simulink model "saturn_thermal4"  (R2021a)
settings: Solver=ode23t  StartTime=0.0  StopTime=80000  MaxStep=1000  RelTol=1e-3
values from neighbouring files (symbols this model uses):
  Ab = L*l    [Data_ini_thermal_analysis4.m]    (also in Data_ini_thermal_analysis5.m)
  As = l*l    [Data_ini_thermal_analysis4.m]    (also in Data_ini_thermal_analysis5.m)
  D_st = 1224526    [Data_ini_thermal_analysis4.m]    (also in Data_ini_thermal_analysis5.m)
  ecc_sc = 0    [Data_ini_thermal_analysis4.m]    (also in Data_ini_thermal_analysis5.m)
  ecc_t = 0.0293    [Data_ini_thermal_analysis4.m]    (also in Data_ini_thermal_analysis5.m)
  incl_ax_s = deg2rad(26.73)    [Data_ini_thermal_analysis4.m]    (also in Data_ini_thermal_analysis5.m)
  incl_sc = deg2rad(90+45)    [Data_ini_thermal_analysis4.m]    (also in Data_ini_thermal_analysis5.m)
  incl_t = deg2rad(0.3485)    [Data_ini_thermal_analysis4.m]    (also in Data_ini_thermal_analysis5.m)
  mean_motion_sc = 2*pi/period_sc    [Data_ini_thermal_analysis4.m]    (also in Data_ini_thermal_analysis5.m)
  mean_motion_t = (2*pi)/period_t    (= 4.56068561416e-06)    [Data_ini_thermal_analysis4.m]    (also in Data_ini_thermal_analysis5.m)
  mean_r_s = 1.427*10^9    (= 1427000000)    [Data_ini_thermal_analysis4.m]    (also in Data_ini_thermal_analysis5.m)
  mu_s = 37931187    [Data_ini_thermal_analysis4.m]    (also in Data_ini_thermal_analysis5.m)
  mu_t = 8971.15    [Data_ini_thermal_analysis4.m]    (also in Data_ini_thermal_analysis5.m)
  period_s = 29.45*365*24*3600    (= 928735200)    [Data_ini_thermal_analysis4.m]    (also in Data_ini_thermal_analysis5.m)
  period_t = 15.945421*24*3600    (= 1377684.3744)    [Data_ini_thermal_analysis4.m]    (also in Data_ini_thermal_analysis5.m)
  R_s = diam_s/2    (= 60268)    [Data_ini_thermal_analysis4.m]    (also in Data_ini_thermal_analysis5.m)
  R_t = 2576    [Data_ini_thermal_analysis4.m]    (also in Data_ini_thermal_analysis5.m)
  semajax_sc = 1500+R_t    (= 4076)    [Data_ini_thermal_analysis4.m]    (also in Data_ini_thermal_analysis5.m)
  semajax_t = 1221830    [Data_ini_thermal_analysis4.m]    (also in Data_ini_thermal_analysis5.m)
libraries: fl_lib x283, nesl_utility x27
(part 1 of 3)
settings Model: Creator=dommy  LastModifiedBy=Riccardo
settings SolverCC: ZeroCrossAlgorithm=Adaptive
settings DebuggingCC: IgnoredZcDiagnostic=none

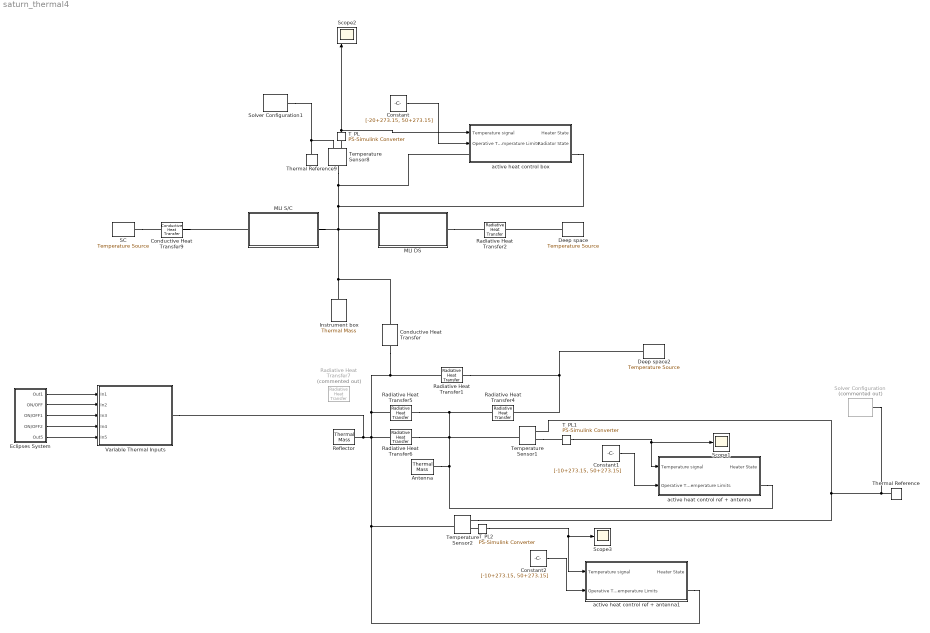
== system saturn_thermal4 ==
  Antenna : fl_lib/Thermal/Thermal Elements/Thermal Mass  mass=m_ant kg  sp_heat=cp_al J/kg/K  T_specify=on  T_priority=High  T=298 K  T_nominal_specify=off  T_nominal_unit=K  T_nominal_value=1  Q_specify=off  Q_priority=None  Q=0 W  Q_nominal_specify=off  Q_nominal_unit=W  Q_nominal_value=1
  Conductive Heat Transfer : fl_lib/Thermal/Thermal Elements/Conductive Heat Transfer  area=A_struc m^2  thickness=0.3 m  th_cond=k_al W/(m*K)  T_specify=off  T_priority=None  T=0 K  T_nominal_specify=off  T_nominal_unit=K  T_nominal_value=1  Q_specify=off  Q_priority=None  Q=0 W  Q_nominal_specify=off  Q_nominal_unit=W  Q_nominal_value=1
  Conductive Heat Transfer9 : fl_lib/Thermal/Thermal Elements/Conductive Heat Transfer  area=2*Ab m^2  thickness=s_kap m  th_cond=k_kap W/(m*K)  T_specify=off  T_priority=None  T=0 K  T_nominal_specify=off  T_nominal_unit=K  T_nominal_value=1  Q_specify=off  Q_priority=None  Q=0 W  Q_nominal_specify=off  Q_nominal_unit=W  Q_nominal_value=1
  Constant : Constant  Value=[-20+273.15, 50+273.15]
  Constant1 : Constant  Value=[-10+273.15, 50+273.15]
  Constant2 : Constant  Value=[-10+273.15, 50+273.15]
  Deep space : fl_lib/Thermal/Thermal Sources/Temperature Source  temperature=T_ds K
  Deep space2 : fl_lib/Thermal/Thermal Sources/Temperature Source  temperature=T_ds K
  Eclipses System : Subsystem
  Instrument box : fl_lib/Thermal/Thermal Elements/Thermal Mass  mass=25 kg  sp_heat=cp_al J/kg/K  T_specify=on  T_priority=High  T=298 K  T_nominal_specify=off  T_nominal_unit=K  T_nominal_value=1  Q_specify=off  Q_priority=None  Q=0 W  Q_nominal_specify=off  Q_nominal_unit=W  Q_nominal_value=1
  MLI DS : Subsystem
  MLI S/C : Subsystem
  Radiative Heat Transfer1 : fl_lib/Thermal/Thermal Elements/Radiative Heat Transfer  area=A_ref m^2  rad_tr_coeff=Gr_al W/(m^2*K^4)  T_specify=off  T_priority=None  T=0 K  T_nominal_specify=off  T_nominal_unit=K  T_nominal_value=1  Q_specify=off  Q_priority=None  Q=0 W  Q_nominal_specify=off  Q_nominal_unit=W  Q_nominal_value=1
      settings: SourceProductBaseCode=SS  InternalSimscapePortConfiguration="{\"Bottom\":[],\"Left\":[{\"id\":\"A\",\"label\":\"A\",\"type\":\"foundation.thermal.thermal\"}],\"Right\":[{\"id\":\"B\",\"label\":\"B\",\"type\":\"foundation.thermal.thermal\"}],\"Top\":[]}"
  Radiative Heat Transfer2 : fl_lib/Thermal/Thermal Elements/Radiative Heat Transfer  area=2*(Ab+As) m^2  rad_tr_coeff=Gr_kap W/(m^2*K^4)  T_specify=off  T_priority=None  T=0 K  T_nominal_specify=off  T_nominal_unit=K  T_nominal_value=1  Q_specify=off  Q_priority=None  Q=0 W  Q_nominal_specify=off  Q_nominal_unit=W  Q_nominal_value=1
      settings: SourceProductBaseCode=SS  InternalSimscapePortConfiguration="{\"Bottom\":[],\"Left\":[{\"id\":\"A\",\"label\":\"A\",\"type\":\"foundation.thermal.thermal\"}],\"Right\":[{\"id\":\"B\",\"label\":\"B\",\"type\":\"foundation.thermal.thermal\"}],\"Top\":[]}"
  Radiative Heat Transfer4 : fl_lib/Thermal/Thermal Elements/Radiative Heat Transfer  area=A_ant m^2  rad_tr_coeff=Gr_al W/(m^2*K^4)  T_specify=off  T_priority=None  T=0 K  T_nominal_specify=off  T_nominal_unit=K  T_nominal_value=1  Q_specify=off  Q_priority=None  Q=0 W  Q_nominal_specify=off  Q_nominal_unit=W  Q_nominal_value=1
      settings: SourceProductBaseCode=SS  InternalSimscapePortConfiguration="{\"Bottom\":[],\"Left\":[{\"id\":\"A\",\"label\":\"A\",\"type\":\"foundation.thermal.thermal\"}],\"Right\":[{\"id\":\"B\",\"label\":\"B\",\"type\":\"foundation.thermal.thermal\"}],\"Top\":[]}"
  Radiative Heat Transfer5 : fl_lib/Thermal/Thermal Elements/Radiative Heat Transfer  area=A_ref m^2  rad_tr_coeff=Gr_ra W/(m^2*K^4)  T_specify=off  T_priority=None  T=0 K  T_nominal_specify=off  T_nominal_unit=K  T_nominal_value=1  Q_specify=off  Q_priority=None  Q=0 W  Q_nominal_specify=off  Q_nominal_unit=W  Q_nominal_value=1
      settings: SourceProductBaseCode=SS  InternalSimscapePortConfiguration="{\"Bottom\":[],\"Left\":[{\"id\":\"A\",\"label\":\"A\",\"type\":\"foundation.thermal.thermal\"}],\"Right\":[{\"id\":\"B\",\"label\":\"B\",\"type\":\"foundation.thermal.thermal\"}],\"Top\":[]}"
  Radiative Heat Transfer6 : fl_lib/Thermal/Thermal Elements/Radiative Heat Transfer  area=A_ant m^2  rad_tr_coeff=Gr_ar W/(m^2*K^4)  T_specify=off  T_priority=None  T=0 K  T_nominal_specify=off  T_nominal_unit=K  T_nominal_value=1  Q_specify=off  Q_priority=None  Q=0 W  Q_nominal_specify=off  Q_nominal_unit=W  Q_nominal_value=1
      settings: SourceProductBaseCode=SS  InternalSimscapePortConfiguration="{\"Bottom\":[],\"Left\":[{\"id\":\"A\",\"label\":\"A\",\"type\":\"foundation.thermal.thermal\"}],\"Right\":[{\"id\":\"B\",\"label\":\"B\",\"type\":\"foundation.thermal.thermal\"}],\"Top\":[]}"
  Radiative Heat Transfer7 : fl_lib/Thermal/Thermal Elements/Radiative Heat Transfer  Commented=on  area=A_ref m^2  rad_tr_coeff=Gr_ra W/(m^2*K^4)  T_specify=off  T_priority=None  T=0 K  T_nominal_specify=off  T_nominal_unit=K  T_nominal_value=1  Q_specify=off  Q_priority=None  Q=0 W  Q_nominal_specify=off  Q_nominal_unit=W  Q_nominal_value=1
      settings: SourceProductBaseCode=SS  InternalSimscapePortConfiguration="{\"Bottom\":[],\"Left\":[{\"id\":\"A\",\"label\":\"A\",\"type\":\"foundation.thermal.thermal\"}],\"Right\":[{\"id\":\"B\",\"label\":\"B\",\"type\":\"foundation.thermal.thermal\"}],\"Top\":[]}"
  Reflector : fl_lib/Thermal/Thermal Elements/Thermal Mass  mass=m_ref kg  sp_heat=cp_al J/kg/K  T_specify=on  T_priority=High  T=298 K  T_nominal_specify=off  T_nominal_unit=K  T_nominal_value=1  Q_specify=off  Q_priority=None  Q=0 W  Q_nominal_specify=off  Q_nominal_unit=W  Q_nominal_value=1
  SC : fl_lib/Thermal/Thermal Sources/Temperature Source  temperature=300 K
  Scope1 : Scope
  Scope2 : Scope  NumInputPorts=3
  Scope3 : Scope
  Solver Configuration : nesl_utility/Solver Configuration  Commented=on  PhysicalDomain=network_engine_domain  SubClassName=solver  LeftPortType=input  RightPortType=generic  Tones=[]  Harmonics=[]  SimulateNoise=off  Profile=off  UseLocalSampling=off  EnableSwitchedLinearOptims=on  FrequencyDomain=off  UseCCode=off  RelTol=0.001  AbsTol=1e-06  MinStep=1e-09  ToWorkspace=off  RevertToSquareIcSolve=off  NumHomotopyIterations=100  PhasorMode=off  PhasorModeNumHarmonics=1  DoDC=off  ResidualTolerance=1e-09  UseLocalSolver=off  LocalSolverChoice=NE_BACKWARD_EULER_ADVANCER  LocalSolverSampleTime=0.001  DoFixedCost=off  MaxNonlinIter=3  MaxModeIter=2  ComputeImpulses=off  ImpulseIterations=2  LinearAlgebra=auto  EquationFormulation=NE_TIME_EF  DelaysMemoryBudget=1024  AutomaticFiltering=on  FilteringTimeConstant=0.001  PartitionStorageMethod=AS_NEEDED  PartitionMemoryBudget=1024  PartitionMethod=ROBUST
      settings: SourceProductBaseCode=PW,SS
  Solver Configuration1 : nesl_utility/Solver Configuration  PhysicalDomain=network_engine_domain  SubClassName=solver  LeftPortType=input  RightPortType=generic  Tones=[]  Harmonics=[]  SimulateNoise=off  Profile=off  UseLocalSampling=off  EnableSwitchedLinearOptims=on  FrequencyDomain=off  UseCCode=off  RelTol=0.001  AbsTol=1e-06  MinStep=1e-09  ToWorkspace=off  RevertToSquareIcSolve=off  NumHomotopyIterations=100  PhasorMode=off  PhasorModeNumHarmonics=1  DoDC=off  ResidualTolerance=1e-09  UseLocalSolver=off  LocalSolverChoice=NE_BACKWARD_EULER_ADVANCER  LocalSolverSampleTime=0.001  DoFixedCost=off  MaxNonlinIter=3  MaxModeIter=2  ComputeImpulses=off  ImpulseIterations=2  LinearAlgebra=auto  EquationFormulation=NE_TIME_EF  DelaysMemoryBudget=1024  AutomaticFiltering=on  FilteringTimeConstant=0.001  PartitionStorageMethod=AS_NEEDED  PartitionMemoryBudget=1024  PartitionMethod=ROBUST
      settings: SourceProductBaseCode=PW,SS
  T_PL : nesl_utility/PS-Simulink Converter  PhysicalDomain=network_engine_domain  SubClassName=ps_output  LeftPortType=input  RightPortType=output  PseudoPeriodic=off  Frequencies=[]  Unit=inherit  AffineConversion=off
      settings: SourceProductBaseCode=PW,SS
  T_PL1 : nesl_utility/PS-Simulink Converter  PhysicalDomain=network_engine_domain  SubClassName=ps_output  LeftPortType=input  RightPortType=output  PseudoPeriodic=off  Frequencies=[]  Unit=inherit  AffineConversion=off
      settings: SourceProductBaseCode=PW,SS
  T_PL2 : nesl_utility/PS-Simulink Converter  PhysicalDomain=network_engine_domain  SubClassName=ps_output  LeftPortType=input  RightPortType=output  PseudoPeriodic=off  Frequencies=[]  Unit=inherit  AffineConversion=off
      settings: SourceProductBaseCode=PW,SS
  Temperature Sensor1 : fl_lib/Thermal/Thermal Sensors/Temperature Sensor
  Temperature Sensor2 : fl_lib/Thermal/Thermal Sensors/Temperature Sensor
  Temperature Sensor8 : fl_lib/Thermal/Thermal Sensors/Temperature Sensor
  Thermal Reference : fl_lib/Thermal/Thermal Elements/Thermal Reference
  Thermal Reference9 : fl_lib/Thermal/Thermal Elements/Thermal Reference
  Variable Thermal Inputs : Subsystem
  active heat control box : Subsystem
  active heat control ref + antenna : Subsystem
  active heat control ref + antenna1 : Subsystem
  wires:
  Eclipses System/2(ON/OFF) -> Variable Thermal Inputs/2(In2)
  Eclipses System/3(ON/OFF1) -> Variable Thermal Inputs/3(In3)
  T_PL/1 -> Scope2/1, active heat control box/1(Temperature signal)
  Eclipses System/5(Out5) -> Variable Thermal Inputs/5(In5)
  Eclipses System/1(Out1) -> Variable Thermal Inputs/1(In1)
  Eclipses System/4(ON/OFF2) -> Variable Thermal Inputs/4(In4)
  T_PL1/1 -> Scope1/1, active heat control ref + antenna/1(Temperature signal)
  T_PL2/1 -> active heat control ref + antenna1/1(Temperature signal), Scope3/1
  Constant/1 -> active heat control box/2(Operative Temperature Limits)
  Constant1/1 -> active heat control ref + antenna/2(Operative Temperature Limits)
  Constant2/1 -> active heat control ref + antenna1/2(Operative Temperature Limits)
  connections:
  MLI DS/RConn1 -- Radiative Heat Transfer2/LConn1
  Temperature Sensor8/RConn1 -- Thermal Reference9/LConn1 -- Solver Configuration1/RConn1
  Temperature Sensor8/RConn2 -- T_PL/LConn1
  Deep space/LConn1 -- Radiative Heat Transfer2/RConn1
  Radiative Heat Transfer1/RConn1 -- Radiative Heat Transfer4/RConn1 -- Deep space2/LConn1
  SC/LConn1 -- Conductive Heat Transfer9/LConn1
  Conductive Heat Transfer9/RConn1 -- MLI S/C/RConn1
  Antenna/LConn1 -- Radiative Heat Transfer5/RConn1 -- Radiative Heat Transfer4/LConn1 -- Radiative Heat Transfer6/LConn1 -- Temperature Sensor1/LConn1 -- active heat control ref + antenna/RConn1
  Temperature Sensor1/RConn2 -- T_PL1/LConn1
  Thermal Reference/LConn1 -- Temperature Sensor2/RConn1 -- Temperature Sensor1/RConn1 -- Solver Configuration/RConn1
  Temperature Sensor2/RConn2 -- T_PL2/LConn1
  Instrument box/LConn1 -- Conductive Heat Transfer/RConn1 -- active heat control box/RConn1 -- active heat control box/LConn1 -- Temperature Sensor8/LConn1 -- MLI S/C/LConn1 -- MLI DS/LConn1
  Reflector/LConn1 -- Variable Thermal Inputs/RConn1 -- Radiative Heat Transfer6/RConn1 -- Conductive Heat Transfer/LConn1 -- Radiative Heat Transfer1/LConn1 -- Radiative Heat Transfer5/LConn1 -- Temperature Sensor2/LConn1 -- active heat control ref + antenna1/RConn1

== system saturn_thermal4/Eclipses System ==
  Add : Sum
  Constant : Constant  Value=0
  Saturn-Titan-SC : Subsystem
  Sun-Saturn-Titan : Subsystem
  Sun-Titan-SC : Subsystem
  Out1 : Outport
  ON/OFF : Outport  Port=2
  ON/OFF1 : Outport  Port=3
  ON/OFF2 : Outport  Port=4
  Out5 : Outport  Port=5
  wires:
  Sun-Titan-SC/1(ON/OFF) -> ON/OFF1/1, Add/2
  Constant/1 -> Out5/1
  Saturn-Titan-SC/1(ON/OFF) -> ON/OFF2/1
  Sun-Saturn-Titan/1(ON/OFF) -> ON/OFF/1, Add/1
  Add/1 -> Out1/1

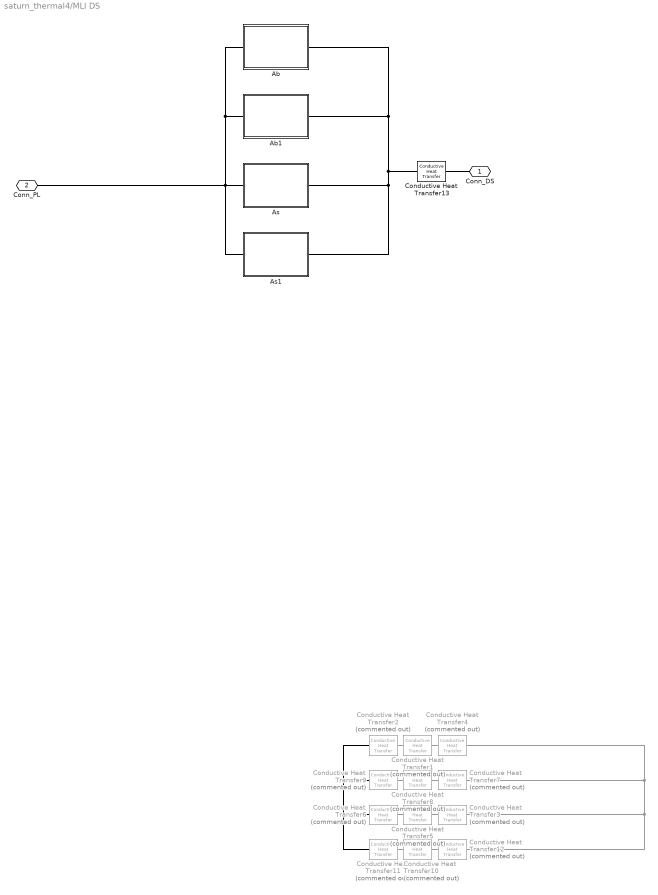
== system saturn_thermal4/MLI DS ==
  Ab : Subsystem
  Ab1 : Subsystem
  As : Subsystem
  As1 : Subsystem
  Conductive Heat Transfer1 : fl_lib/Thermal/Thermal Elements/Conductive Heat Transfer  Commented=on  area=As m^2  thickness=s_tfe_out m  th_cond=k_tfe W/(m*K)  T_specify=off  T_priority=None  T=0 K  T_nominal_specify=off  T_nominal_unit=K  T_nominal_value=1  Q_specify=off  Q_priority=None  Q=0 W  Q_nominal_specify=off  Q_nominal_unit=W  Q_nominal_value=1
  Conductive Heat Transfer10 : fl_lib/Thermal/Thermal Elements/Conductive Heat Transfer  Commented=on  area=As m^2  thickness=s_tfe_out m  th_cond=k_tfe W/(m*K)  T_specify=off  T_priority=None  T=0 K  T_nominal_specify=off  T_nominal_unit=K  T_nominal_value=1  Q_specify=off  Q_priority=None  Q=0 W  Q_nominal_specify=off  Q_nominal_unit=W  Q_nominal_value=1
  Conductive Heat Transfer{2,4,11..12} (4 alike) : fl_lib/Thermal/Thermal Elements/Conductive Heat Transfer  Commented=on  area=As m^2  thickness=s_al m  th_cond=k_al W/(m*K)  T_specify=off  T_priority=None  T=0 K  T_nominal_specify=off  T_nominal_unit=K  T_nominal_value=1  Q_specify=off  Q_priority=None  Q=0 W  Q_nominal_specify=off  Q_nominal_unit=W  Q_nominal_value=1
  Conductive Heat Transfer13 : fl_lib/Thermal/Thermal Elements/Conductive Heat Transfer  area=2*(Ab+As) m^2  thickness=s_kap m  th_cond=k_kap W/(m*K)  T_specify=off  T_priority=None  T=0 K  T_nominal_specify=off  T_nominal_unit=K  T_nominal_value=1  Q_specify=off  Q_priority=None  Q=0 W  Q_nominal_specify=off  Q_nominal_unit=W  Q_nominal_value=1
  Conductive Heat Transfer{3,6..7,9} (4 alike) : fl_lib/Thermal/Thermal Elements/Conductive Heat Transfer  Commented=on  area=Ab m^2  thickness=s_al m  th_cond=k_al W/(m*K)  T_specify=off  T_priority=None  T=0 K  T_nominal_specify=off  T_nominal_unit=K  T_nominal_value=1  Q_specify=off  Q_priority=None  Q=0 W  Q_nominal_specify=off  Q_nominal_unit=W  Q_nominal_value=1
  Conductive Heat Transfer5 : fl_lib/Thermal/Thermal Elements/Conductive Heat Transfer  Commented=on  area=Ab m^2  thickness=s_tfe_out m  th_cond=k_tfe W/(m*K)  T_specify=off  T_priority=None  T=0 K  T_nominal_specify=off  T_nominal_unit=K  T_nominal_value=1  Q_specify=off  Q_priority=None  Q=0 W  Q_nominal_specify=off  Q_nominal_unit=W  Q_nominal_value=1
  Conductive Heat Transfer8 : fl_lib/Thermal/Thermal Elements/Conductive Heat Transfer  Commented=on  area=Ab m^2  thickness=s_tfe_out m  th_cond=k_tfe W/(m*K)  T_specify=off  T_priority=None  T=0 K  T_nominal_specify=off  T_nominal_unit=K  T_nominal_value=1  Q_specify=off  Q_priority=None  Q=0 W  Q_nominal_specify=off  Q_nominal_unit=W  Q_nominal_value=1
  Conn_DS : PMIOPort  Side=Right
  "Conn_PL\t" : PMIOPort  Port=2  Side=Left
  connections:
  Conductive Heat Transfer7/RConn1 -- Conductive Heat Transfer3/RConn1 -- Conductive Heat Transfer12/RConn1 -- Conductive Heat Transfer4/RConn1
  Conductive Heat Transfer11/RConn1 -- Conductive Heat Transfer10/LConn1
  Conductive Heat Transfer12/LConn1 -- Conductive Heat Transfer10/RConn1
  Conductive Heat Transfer6/RConn1 -- Conductive Heat Transfer5/LConn1
  Conductive Heat Transfer3/LConn1 -- Conductive Heat Transfer5/RConn1
  Conductive Heat Transfer7/LConn1 -- Conductive Heat Transfer8/RConn1
  Conductive Heat Transfer9/RConn1 -- Conductive Heat Transfer8/LConn1
  Conductive Heat Transfer4/LConn1 -- Conductive Heat Transfer1/RConn1
  Conductive Heat Transfer2/RConn1 -- Conductive Heat Transfer1/LConn1
  Conductive Heat Transfer9/LConn1 -- Conductive Heat Transfer11/LConn1 -- Conductive Heat Transfer6/LConn1 -- Conductive Heat Transfer2/LConn1
  "Conn_PL\t"/RConn1 -- Ab/LConn1 -- Ab1/LConn1 -- As/LConn1 -- As1/LConn1
  Conn_DS/RConn1 -- Conductive Heat Transfer13/RConn1
  Conductive Heat Transfer13/LConn1 -- Ab/RConn1 -- Ab1/RConn1 -- As/RConn1 -- As1/RConn1

== system saturn_thermal4/MLI S//C ==
  Ab : Subsystem
  Ab1 : Subsystem
  Conductive Heat Transfer1 : fl_lib/Thermal/Thermal Elements/Conductive Heat Transfer  Commented=on  area=As m^2  thickness=s_tfe_out m  th_cond=k_tfe W/(m*K)  T_specify=off  T_priority=None  T=0 K  T_nominal_specify=off  T_nominal_unit=K  T_nominal_value=1  Q_specify=off  Q_priority=None  Q=0 W  Q_nominal_specify=off  Q_nominal_unit=W  Q_nominal_value=1
  Conductive Heat Transfer10 : fl_lib/Thermal/Thermal Elements/Conductive Heat Transfer  Commented=on  area=As m^2  thickness=s_tfe_out m  th_cond=k_tfe W/(m*K)  T_specify=off  T_priority=None  T=0 K  T_nominal_specify=off  T_nominal_unit=K  T_nominal_value=1  Q_specify=off  Q_priority=None  Q=0 W  Q_nominal_specify=off  Q_nominal_unit=W  Q_nominal_value=1
  Conductive Heat Transfer{2,4,11..12} (4 alike) : fl_lib/Thermal/Thermal Elements/Conductive Heat Transfer  Commented=on  area=As m^2  thickness=s_al m  th_cond=k_al W/(m*K)  T_specify=off  T_priority=None  T=0 K  T_nominal_specify=off  T_nominal_unit=K  T_nominal_value=1  Q_specify=off  Q_priority=None  Q=0 W  Q_nominal_specify=off  Q_nominal_unit=W  Q_nominal_value=1
  Conductive Heat Transfer{3,6..7,9} (4 alike) : fl_lib/Thermal/Thermal Elements/Conductive Heat Transfer  Commented=on  area=Ab m^2  thickness=s_al m  th_cond=k_al W/(m*K)  T_specify=off  T_priority=None  T=0 K  T_nominal_specify=off  T_nominal_unit=K  T_nominal_value=1  Q_specify=off  Q_priority=None  Q=0 W  Q_nominal_specify=off  Q_nominal_unit=W  Q_nominal_value=1
  Conductive Heat Transfer5 : fl_lib/Thermal/Thermal Elements/Conductive Heat Transfer  Commented=on  area=Ab m^2  thickness=s_tfe_out m  th_cond=k_tfe W/(m*K)  T_specify=off  T_priority=None  T=0 K  T_nominal_specify=off  T_nominal_unit=K  T_nominal_value=1  Q_specify=off  Q_priority=None  Q=0 W  Q_nominal_specify=off  Q_nominal_unit=W  Q_nominal_value=1
  Conductive Heat Transfer8 : fl_lib/Thermal/Thermal Elements/Conductive Heat Transfer  Commented=on  area=Ab m^2  thickness=s_tfe_out m  th_cond=k_tfe W/(m*K)  T_specify=off  T_priority=None  T=0 K  T_nominal_specify=off  T_nominal_unit=K  T_nominal_value=1  Q_specify=off  Q_priority=None  Q=0 W  Q_nominal_specify=off  Q_nominal_unit=W  Q_nominal_value=1
  Conn_S/C : PMIOPort  Side=Right
  "Conn_PL\t" : PMIOPort  Port=2  Side=Left
  connections:
  Ab1/RConn1 -- Ab/RConn1 -- Conn_S/C/RConn1
  Ab1/LConn1 -- Ab/LConn1 -- "Conn_PL\t"/RConn1
  Conductive Heat Transfer2/LConn1 -- Conductive Heat Transfer6/LConn1 -- Conductive Heat Transfer11/LConn1 -- Conductive Heat Transfer9/LConn1
  Conductive Heat Transfer2/RConn1 -- Conductive Heat Transfer1/LConn1
  Conductive Heat Transfer4/LConn1 -- Conductive Heat Transfer1/RConn1
  Conductive Heat Transfer9/RConn1 -- Conductive Heat Transfer8/LConn1
  Conductive Heat Transfer7/LConn1 -- Conductive Heat Transfer8/RConn1
  Conductive Heat Transfer3/LConn1 -- Conductive Heat Transfer5/RConn1
  Conductive Heat Transfer6/RConn1 -- Conductive Heat Transfer5/LConn1
  Conductive Heat Transfer12/LConn1 -- Conductive Heat Transfer10/RConn1
  Conductive Heat Transfer11/RConn1 -- Conductive Heat Transfer10/LConn1
  Conductive Heat Transfer4/RConn1 -- Conductive Heat Transfer12/RConn1 -- Conductive Heat Transfer3/RConn1 -- Conductive Heat Transfer7/RConn1

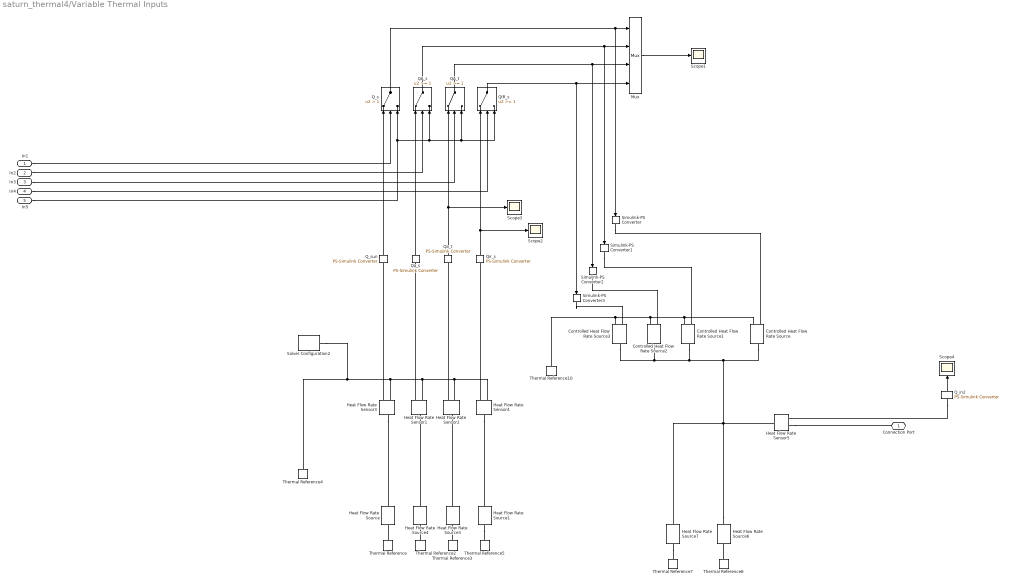
== system saturn_thermal4/Variable Thermal Inputs ==
  In1 : Inport
  In2 : Inport  Port=2
  In3 : Inport  Port=3
  In4 : Inport  Port=4
  In5 : Inport  Port=5
  Controlled Heat Flow Rate Source{,1..3} (4 alike) : fl_lib/Thermal/Thermal Sources/Controlled Heat Flow Rate Source
  Heat Flow Rate Sensor{1..5} (5 alike) : fl_lib/Thermal/Thermal Sensors/Heat Flow Rate Sensor
      settings: SourceProductBaseCode=SS
  Heat Flow Rate Source : fl_lib/Thermal/Thermal Sources/Heat Flow Rate Source  heat_flow=Qs_s W
      settings: SourceProductBaseCode=SS  InternalSimscapePortConfiguration="{\"Bottom\":[],\"Left\":[{\"id\":\"B\",\"label\":\"B\",\"type\":\"foundation.thermal.thermal\"}],\"Right\":[{\"id\":\"A\",\"label\":\"A\",\"type\":\"foundation.thermal.thermal\"}],\"Top\":[]}"
  Heat Flow Rate Source1 : fl_lib/Thermal/Thermal Sources/Heat Flow Rate Source  heat_flow=Qir_s W
      settings: SourceProductBaseCode=SS  InternalSimscapePortConfiguration="{\"Bottom\":[],\"Left\":[{\"id\":\"B\",\"label\":\"B\",\"type\":\"foundation.thermal.thermal\"}],\"Right\":[{\"id\":\"A\",\"label\":\"A\",\"type\":\"foundation.thermal.thermal\"}],\"Top\":[]}"
  Heat Flow Rate Source3 : fl_lib/Thermal/Thermal Sources/Heat Flow Rate Source  heat_flow=Qa_t W
      settings: SourceProductBaseCode=SS  InternalSimscapePortConfiguration="{\"Bottom\":[],\"Left\":[{\"id\":\"B\",\"label\":\"B\",\"type\":\"foundation.thermal.thermal\"}],\"Right\":[{\"id\":\"A\",\"label\":\"A\",\"type\":\"foundation.thermal.thermal\"}],\"Top\":[]}"
  Heat Flow Rate Source4 : fl_lib/Thermal/Thermal Sources/Heat Flow Rate Source  heat_flow=Qa_s W
      settings: SourceProductBaseCode=SS  InternalSimscapePortConfiguration="{\"Bottom\":[],\"Left\":[{\"id\":\"B\",\"label\":\"B\",\"type\":\"foundation.thermal.thermal\"}],\"Right\":[{\"id\":\"A\",\"label\":\"A\",\"type\":\"foundation.thermal.thermal\"}],\"Top\":[]}"
  Heat Flow Rate Source6 : fl_lib/Thermal/Thermal Sources/Heat Flow Rate Source  heat_flow=45 W
      settings: SourceProductBaseCode=SS  InternalSimscapePortConfiguration="{\"Bottom\":[],\"Left\":[{\"id\":\"B\",\"label\":\"B\",\"type\":\"foundation.thermal.thermal\"}],\"Right\":[{\"id\":\"A\",\"label\":\"A\",\"type\":\"foundation.thermal.thermal\"}],\"Top\":[]}"
  Heat Flow Rate Source7 : fl_lib/Thermal/Thermal Sources/Heat Flow Rate Source  heat_flow=Qir_t W
      settings: SourceProductBaseCode=SS  InternalSimscapePortConfiguration="{\"Bottom\":[],\"Left\":[{\"id\":\"B\",\"label\":\"B\",\"type\":\"foundation.thermal.thermal\"}],\"Right\":[{\"id\":\"A\",\"label\":\"A\",\"type\":\"foundation.thermal.thermal\"}],\"Top\":[]}"
  Mux : Mux
  QA_s : Switch  Threshold=1
  QA_t : Switch  Threshold=1
  QIR_s : Switch  Threshold=1
  Q_in2 : nesl_utility/PS-Simulink Converter  PhysicalDomain=network_engine_domain  SubClassName=ps_output  LeftPortType=input  RightPortType=output  PseudoPeriodic=off  Frequencies=[]  Unit=inherit  AffineConversion=off
      settings: SourceProductBaseCode=PW,SS
  Q_s : Switch  Criteria=u2 > Threshold  Threshold=1
  Q_sun : nesl_utility/PS-Simulink Converter  PhysicalDomain=network_engine_domain  SubClassName=ps_output  LeftPortType=input  RightPortType=output  PseudoPeriodic=off  Frequencies=[]  Unit=inherit  AffineConversion=off
      settings: SourceProductBaseCode=PW,SS
  Qa_s : nesl_utility/PS-Simulink Converter  PhysicalDomain=network_engine_domain  SubClassName=ps_output  LeftPortType=input  RightPortType=output  PseudoPeriodic=off  Frequencies=[]  Unit=inherit  AffineConversion=off
      settings: SourceProductBaseCode=PW,SS
  Qa_t : nesl_utility/PS-Simulink Converter  PhysicalDomain=network_engine_domain  SubClassName=ps_output  LeftPortType=input  RightPortType=output  PseudoPeriodic=off  Frequencies=[]  Unit=inherit  AffineConversion=off
      settings: SourceProductBaseCode=PW,SS
  Qir_s : nesl_utility/PS-Simulink Converter  PhysicalDomain=network_engine_domain  SubClassName=ps_output  LeftPortType=input  RightPortType=output  PseudoPeriodic=off  Frequencies=[]  Unit=inherit  AffineConversion=off
      settings: SourceProductBaseCode=PW,SS
  Scope{1..4} (4 alike) : Scope
  Simulink-PS Converter{,1..3} (4 alike) : nesl_utility/Simulink-PS Converter  PhysicalDomain=network_engine_domain  SubClassName=ps_input  LeftPortType=input  RightPortType=output  PseudoPeriodic=off  Frequencies=[]  NoiseDistribution=none  NoiseParameters=[]  Unit=1  AffineConversion=off  FilteringAndDerivatives=provide  SimscapeFilterOrder=1  InputFilterTimeConstant=0.001  UdotUserProvided=0
      settings: SourceProductBaseCode=PW,SS
  Solver Configuration2 : nesl_utility/Solver Configuration  PhysicalDomain=network_engine_domain  SubClassName=solver  LeftPortType=input  RightPortType=generic  Tones=[]  Harmonics=[]  SimulateNoise=off  Profile=off  UseLocalSampling=off  EnableSwitchedLinearOptims=on  FrequencyDomain=off  UseCCode=off  RelTol=0.001  AbsTol=1e-06  MinStep=1e-09  ToWorkspace=off  RevertToSquareIcSolve=off  NumHomotopyIterations=100  PhasorMode=off  PhasorModeNumHarmonics=1  DoDC=off  ResidualTolerance=1e-09  UseLocalSolver=off  LocalSolverChoice=NE_BACKWARD_EULER_ADVANCER  LocalSolverSampleTime=0.001  DoFixedCost=off  MaxNonlinIter=3  MaxModeIter=2  ComputeImpulses=off  ImpulseIterations=2  LinearAlgebra=auto  EquationFormulation=NE_TIME_EF  DelaysMemoryBudget=1024  AutomaticFiltering=on  FilteringTimeConstant=0.001  PartitionStorageMethod=AS_NEEDED  PartitionMemoryBudget=1024  PartitionMethod=ROBUST
      settings: SourceProductBaseCode=PW,SS
  Thermal Reference{,2..5,7..8,10} (8 alike) : fl_lib/Thermal/Thermal Elements/Thermal Reference
  Connection Port : PMIOPort  Side=Right
  wires:
  QA_t/1 -> Simulink-PS Converter2/1, Mux/3
  In5/1 -> QA_s/3, QIR_s/3, QA_t/3, Q_s/3
  Qa_s/1 -> QA_s/1
  QIR_s/1 -> Simulink-PS Converter3/1, Mux/4
  QA_s/1 -> Simulink-PS Converter1/1, Mux/2
  Qa_t/1 -> Scope3/1, QA_t/1
  Q_sun/1 -> Q_s/1
  Q_s/1 -> Simulink-PS Converter/1, Mux/1
  Qir_s/1 -> QIR_s/1, Scope2/1
  Mux/1 -> Scope1/1
  In4/1 -> QIR_s/2
  In2/1 -> QA_s/2
  In1/1 -> Q_s/2
  In3/1 -> QA_t/2
  Q_in2/1 -> Scope4/1
  connections:
  Thermal Reference4/LConn1 -- Solver Configuration2/RConn1 -- Heat Flow Rate Sensor3/RConn2 -- Heat Flow Rate Sensor1/RConn2 -- Heat Flow Rate Sensor2/RConn2 -- Heat Flow Rate Sensor4/RConn2
  Thermal Reference8/LConn1 -- Heat Flow Rate Source6/RConn1
  Heat Flow Rate Sensor1/LConn1 -- Heat Flow Rate Source4/LConn1
  Heat Flow Rate Source4/RConn1 -- Thermal Reference2/LConn1
  Thermal Reference10/LConn1 -- Controlled Heat Flow Rate Source3/RConn2 -- Controlled Heat Flow Rate Source/RConn2 -- Controlled Heat Flow Rate Source1/RConn2 -- Controlled Heat Flow Rate Source2/RConn2
  Thermal Reference3/LConn1 -- Heat Flow Rate Source3/RConn1
  Heat Flow Rate Source1/RConn1 -- Thermal Reference5/LConn1
  Heat Flow Rate Sensor2/RConn1 -- Qa_t/LConn1
  Thermal Reference/LConn1 -- Heat Flow Rate Source/RConn1
  Simulink-PS Converter1/RConn1 -- Controlled Heat Flow Rate Source1/RConn1
  Simulink-PS Converter2/RConn1 -- Controlled Heat Flow Rate Source2/RConn1
  Simulink-PS Converter3/RConn1 -- Controlled Heat Flow Rate Source3/RConn1
  Heat Flow Rate Sensor1/RConn1 -- Qa_s/LConn1
  Heat Flow Rate Sensor4/RConn1 -- Qir_s/LConn1
  Heat Flow Rate Source7/RConn1 -- Thermal Reference7/LConn1
  Simulink-PS Converter/RConn1 -- Controlled Heat Flow Rate Source/RConn1
  Heat Flow Rate Sensor3/RConn1 -- Q_sun/LConn1
  Heat Flow Rate Sensor4/LConn1 -- Heat Flow Rate Source1/LConn1
  Heat Flow Rate Sensor2/LConn1 -- Heat Flow Rate Source3/LConn1
  Heat Flow Rate Sensor3/LConn1 -- Heat Flow Rate Source/LConn1
  Q_in2/LConn1 -- Heat Flow Rate Sensor5/RConn1
  Heat Flow Rate Source6/LConn1 -- Heat Flow Rate Sensor5/LConn1 -- Heat Flow Rate Source7/LConn1 -- Controlled Heat Flow Rate Source/LConn1 -- Controlled Heat Flow Rate Source3/LConn1 -- Controlled Heat Flow Rate Source2/LConn1 -- Controlled Heat Flow Rate Source1/LConn1
  Heat Flow Rate Sensor5/RConn2 -- Connection Port/RConn1

== system saturn_thermal4/active heat control box ==
  Temperature signal : Inport
  Operative Temperature Limits : Inport  Port=2
  Constant : Constant  Value=0
  Demux : Demux  Outputs=2
  Heater Watts : Constant  Value=50
  Subsystem : Subsystem
  Subsystem1 : Subsystem
      settings: PortSchema="{\"entries\":[{\"content\":{\"sides\":[{\"content\":{\"connectorIds\":[\"In1\",\"LConn1\",\"In2\",\"In3\"]},\"type\":\"ConnectorPlacement.EquallySpacedRectSide\",\"uuid\":\"bd26e488-957e-4768-8c8f-f592c40ec45a\"},{\"content\":{\"connectorIds\":[\"Out1\"],\"side\":\"RIGHT\"},\"type\":\"ConnectorPlacement.EquallySpacedRectSide\",\"uuid\":\"e3290ae6-0dd6-4908-9dc2-c69eb2f26011\"},{\"content\":{\"connectorIds\":[],\"side\":\"TOP\"},\"type\":\"ConnectorPlacement.EquallySpacedRectSide\",\"uuid\":\"6f74d5de-8d2d-4ebd-b7f8-350d8117613a\"}]},\"type\":\"ConnectorPlacement.EquallySpacedConnector\",\"uuid\":\"06df4fc0-1d31-4bf7-986e-18508187f506\"}],\"packageUris\":[\"http://schema.mathworks.com/mf0/Connector/R2020b\"],\"version\":\"1.0\"}"
  heat block : PMIOPort  Side=Left
  Heater Sink : PMIOPort  Port=2  Side=Right
  Heater State : Outport
  Radiator State : Outport  Port=2
  wires:
  Temperature signal/1 -> Subsystem1/1(signal), Subsystem/1(signal)
  Operative Temperature Limits/1 -> Demux/1
  Demux/1 -> Subsystem/2(reference)
  Demux/2 -> Subsystem1/2(reference)
  Constant/1 -> Subsystem/4(off case), Subsystem1/3(off case)
  Heater Watts/1 -> Subsystem/3(on case)
  Subsystem/1(Output) -> Heater State/1
  Subsystem1/1(Output) -> Radiator State/1
  connections:
  heat block/RConn1 -- Subsystem1/LConn1
  Heater Sink/RConn1 -- Subsystem/RConn1

== system saturn_thermal4/active heat control ref + antenna ==
  Temperature signal : Inport
  Operative Temperature Limits : Inport  Port=2
  Constant : Constant  Value=0
  Demux : Demux  Outputs=2
  Heater Watts : Constant  Value=50
  Subsystem : Subsystem
  Subsystem1 : Subsystem  Commented=on
      settings: PortSchema="{\"entries\":[{\"content\":{\"sides\":[{\"content\":{\"connectorIds\":[\"In1\",\"LConn1\",\"In2\",\"In3\"]},\"type\":\"ConnectorPlacement.EquallySpacedRectSide\",\"uuid\":\"bd26e488-957e-4768-8c8f-f592c40ec45a\"},{\"content\":{\"connectorIds\":[\"Out1\"],\"side\":\"RIGHT\"},\"type\":\"ConnectorPlacement.EquallySpacedRectSide\",\"uuid\":\"e3290ae6-0dd6-4908-9dc2-c69eb2f26011\"},{\"content\":{\"connectorIds\":[],\"side\":\"TOP\"},\"type\":\"ConnectorPlacement.EquallySpacedRectSide\",\"uuid\":\"6f74d5de-8d2d-4ebd-b7f8-350d8117613a\"}]},\"type\":\"ConnectorPlacement.EquallySpacedConnector\",\"uuid\":\"06df4fc0-1d31-4bf7-986e-18508187f506\"}],\"packageUris\":[\"http://schema.mathworks.com/mf0/Connector/R2020b\"],\"version\":\"1.0\"}"
  Heater Sink : PMIOPort  Side=Right
  Heater State : Outport
  wires:
  Temperature signal/1 -> Subsystem/1(signal)
  Operative Temperature Limits/1 -> Demux/1
  Demux/1 -> Subsystem/2(reference)
  Constant/1 -> Subsystem/4(off case)
  Heater Watts/1 -> Subsystem/3(on case)
  Subsystem/1(Output) -> Heater State/1
  Demux/2 -> Subsystem1/1(signal)
  connections:
  Heater Sink/RConn1 -- Subsystem/RConn1

== system saturn_thermal4/active heat control ref + antenna1 ==
  Temperature signal : Inport
  Operative Temperature Limits : Inport  Port=2
  Constant : Constant  Value=0
  Demux : Demux  Outputs=2
  Heater Watts : Constant  Value=200
  Subsystem : Subsystem
  Subsystem1 : Subsystem  Commented=on
      settings: PortSchema="{\"entries\":[{\"content\":{\"sides\":[{\"content\":{\"connectorIds\":[\"In1\",\"LConn1\",\"In2\",\"In3\"]},\"type\":\"ConnectorPlacement.EquallySpacedRectSide\",\"uuid\":\"bd26e488-957e-4768-8c8f-f592c40ec45a\"},{\"content\":{\"connectorIds\":[\"Out1\"],\"side\":\"RIGHT\"},\"type\":\"ConnectorPlacement.EquallySpacedRectSide\",\"uuid\":\"e3290ae6-0dd6-4908-9dc2-c69eb2f26011\"},{\"content\":{\"connectorIds\":[],\"side\":\"TOP\"},\"type\":\"ConnectorPlacement.EquallySpacedRectSide\",\"uuid\":\"6f74d5de-8d2d-4ebd-b7f8-350d8117613a\"}]},\"type\":\"ConnectorPlacement.EquallySpacedConnector\",\"uuid\":\"06df4fc0-1d31-4bf7-986e-18508187f506\"}],\"packageUris\":[\"http://schema.mathworks.com/mf0/Connector/R2020b\"],\"version\":\"1.0\"}"
  Terminator : Terminator
  Heater Sink : PMIOPort  Side=Right
  Heater State : Outport
  wires:
  Temperature signal/1 -> Subsystem/1(signal)
  Operative Temperature Limits/1 -> Demux/1
  Demux/1 -> Subsystem/2(reference)
  Constant/1 -> Subsystem/4(off case)
  Heater Watts/1 -> Subsystem/3(on case)
  Subsystem/1(Output) -> Heater State/1
  Demux/2 -> Terminator/1
  connections:
  Heater Sink/RConn1 -- Subsystem/RConn1

== system saturn_thermal4/Eclipses System/Saturn-Titan-SC ==
  S/C Titan Saturn : Subsystem
  S/C-Titan orbit : Subsystem
  Titan-Saturn orbit : Subsystem
  ON/OFF : Outport
  wires:
  S/C-Titan orbit/1(r_mn) -> S/C Titan Saturn/2(r_mn)
  Titan-Saturn orbit/1(S_mn) -> S/C Titan Saturn/1(S_mn)
  S/C Titan Saturn/1(ON/OFF) -> ON/OFF/1

== system saturn_thermal4/Eclipses System/Sun-Saturn-Titan ==
  Saturn-Sun orbit : Subsystem
  Titan-Saturn : Subsystem
  Titan-Saturn-Sun Eclipse : Subsystem
  ON/OFF : Outport
  wires:
  Saturn-Sun orbit/1(S_mn) -> Titan-Saturn-Sun Eclipse/1(S_mn)
  Titan-Saturn/1(r_mn) -> Titan-Saturn-Sun Eclipse/2(r_mn)
  Titan-Saturn-Sun Eclipse/1(ON/OFF) -> ON/OFF/1

== system saturn_thermal4/Eclipses System/Sun-Titan-SC ==
  Ecliptic Orbital parameter1 : Subsystem
  Orbit Parameter1 : Subsystem
  S/C Titan Sun Eclipse : Subsystem
  ON/OFF : Outport
  wires:
  Ecliptic Orbital parameter1/1(S_mn) -> S/C Titan Sun Eclipse/1(S_mn)
  Orbit Parameter1/1(r_mn) -> S/C Titan Sun Eclipse/2(r_mn)
  S/C Titan Sun Eclipse/1(ON/OFF) -> ON/OFF/1

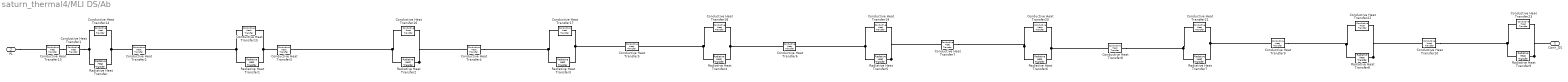
== system saturn_thermal4/MLI DS/Ab ==
  Conductive Heat Transfer{1..10} (10 alike) : fl_lib/Thermal/Thermal Elements/Conductive Heat Transfer  area=Ab m^2  thickness=s_kap m  th_cond=k_kap W/(m*K)  T_specify=off  T_priority=None  T=0 K  T_nominal_specify=off  T_nominal_unit=K  T_nominal_value=1  Q_specify=off  Q_priority=None  Q=0 W  Q_nominal_specify=off  Q_nominal_unit=W  Q_nominal_value=1
  Conductive Heat Transfer13 : fl_lib/Thermal/Thermal Elements/Conductive Heat Transfer  area=Ab m^2  thickness=s_al m  th_cond=k_al W/(m*K)  T_specify=off  T_priority=None  T=0 K  T_nominal_specify=off  T_nominal_unit=K  T_nominal_value=1  Q_specify=off  Q_priority=None  Q=0 W  Q_nominal_specify=off  Q_nominal_unit=W  Q_nominal_value=1
  Conductive Heat Transfer{14..23} (10 alike) : fl_lib/Thermal/Thermal Elements/Conductive Heat Transfer  area=A_net_new_b m^2  thickness=s_tfe_out m  th_cond=k_tfe W/(m*K)  T_specify=off  T_priority=None  T=0 K  T_nominal_specify=off  T_nominal_unit=K  T_nominal_value=1  Q_specify=off  Q_priority=None  Q=0 W  Q_nominal_specify=off  Q_nominal_unit=W  Q_nominal_value=1
  Radiative Heat Transfer{,1..9} (10 alike) : fl_lib/Thermal/Thermal Elements/Radiative Heat Transfer  area=A_empty_b m^2  rad_tr_coeff=Gr_kap_mli W/(m^2*K^4)  T_specify=off  T_priority=None  T=0 K  T_nominal_specify=off  T_nominal_unit=K  T_nominal_value=1  Q_specify=off  Q_priority=None  Q=0 W  Q_nominal_specify=off  Q_nominal_unit=W  Q_nominal_value=1
      settings: SourceProductBaseCode=SS  InternalSimscapePortConfiguration="{\"Bottom\":[],\"Left\":[{\"id\":\"A\",\"label\":\"A\",\"type\":\"foundation.thermal.thermal\"}],\"Right\":[{\"id\":\"B\",\"label\":\"B\",\"type\":\"foundation.thermal.thermal\"}],\"Top\":[]}"
  Conn_DS : PMIOPort  Side=Right
  PL : PMIOPort  Port=2  Side=Left
  connections:
  Conductive Heat Transfer19/LConn1 -- Radiative Heat Transfer5/LConn1 -- Conductive Heat Transfer6/RConn1
  Conductive Heat Transfer20/RConn1 -- Radiative Heat Transfer6/RConn1 -- Conductive Heat Transfer8/LConn1
  Conductive Heat Transfer21/LConn1 -- Radiative Heat Transfer7/LConn1 -- Conductive Heat Transfer8/RConn1
  Conductive Heat Transfer17/LConn1 -- Radiative Heat Transfer3/LConn1 -- Conductive Heat Transfer4/RConn1
  Radiative Heat Transfer5/RConn1 -- Conductive Heat Transfer19/RConn1 -- Conductive Heat Transfer7/LConn1
  Radiative Heat Transfer/LConn1 -- Conductive Heat Transfer1/RConn1 -- Conductive Heat Transfer14/LConn1
  Radiative Heat Transfer4/LConn1 -- Conductive Heat Transfer18/LConn1 -- Conductive Heat Transfer5/RConn1
  Conductive Heat Transfer7/RConn1 -- Conductive Heat Transfer20/LConn1 -- Radiative Heat Transfer6/LConn1
  Conductive Heat Transfer9/LConn1 -- Conductive Heat Transfer21/RConn1 -- Radiative Heat Transfer7/RConn1
  Conductive Heat Transfer18/RConn1 -- Radiative Heat Transfer4/RConn1 -- Conductive Heat Transfer6/LConn1
  Conductive Heat Transfer5/LConn1 -- Conductive Heat Transfer17/RConn1 -- Radiative Heat Transfer3/RConn1
  Radiative Heat Transfer9/LConn1 -- Conductive Heat Transfer23/LConn1 -- Conductive Heat Transfer10/RConn1
  Radiative Heat Transfer/RConn1 -- Conductive Heat Transfer14/RConn1 -- Conductive Heat Transfer2/LConn1
  Radiative Heat Transfer2/LConn1 -- Conductive Heat Transfer16/LConn1 -- Conductive Heat Transfer3/RConn1
  Radiative Heat Transfer2/RConn1 -- Conductive Heat Transfer16/RConn1 -- Conductive Heat Transfer4/LConn1
  Conductive Heat Transfer3/LConn1 -- Conductive Heat Transfer15/RConn1 -- Radiative Heat Transfer1/RConn1
  Radiative Heat Transfer9/RConn1 -- Conductive Heat Transfer23/RConn1 -- Conn_DS/RConn1
  Conductive Heat Transfer15/LConn1 -- Radiative Heat Transfer1/LConn1 -- Conductive Heat Transfer2/RConn1
  Radiative Heat Transfer8/LConn1 -- Conductive Heat Transfer22/LConn1 -- Conductive Heat Transfer9/RConn1
  Radiative Heat Transfer8/RConn1 -- Conductive Heat Transfer22/RConn1 -- Conductive Heat Transfer10/LConn1
  PL/RConn1 -- Conductive Heat Transfer13/LConn1
  Conductive Heat Transfer13/RConn1 -- Conductive Heat Transfer1/LConn1

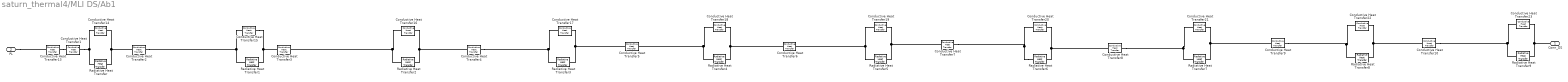
== system saturn_thermal4/MLI DS/Ab1 ==
  Conductive Heat Transfer{1..10} (10 alike) : fl_lib/Thermal/Thermal Elements/Conductive Heat Transfer  area=Ab m^2  thickness=s_kap m  th_cond=k_kap W/(m*K)  T_specify=off  T_priority=None  T=0 K  T_nominal_specify=off  T_nominal_unit=K  T_nominal_value=1  Q_specify=off  Q_priority=None  Q=0 W  Q_nominal_specify=off  Q_nominal_unit=W  Q_nominal_value=1
  Conductive Heat Transfer13 : fl_lib/Thermal/Thermal Elements/Conductive Heat Transfer  area=Ab m^2  thickness=s_al m  th_cond=k_al W/(m*K)  T_specify=off  T_priority=None  T=0 K  T_nominal_specify=off  T_nominal_unit=K  T_nominal_value=1  Q_specify=off  Q_priority=None  Q=0 W  Q_nominal_specify=off  Q_nominal_unit=W  Q_nominal_value=1
  Conductive Heat Transfer{14..23} (10 alike) : fl_lib/Thermal/Thermal Elements/Conductive Heat Transfer  area=A_net_new_b m^2  thickness=s_tfe_out m  th_cond=k_tfe W/(m*K)  T_specify=off  T_priority=None  T=0 K  T_nominal_specify=off  T_nominal_unit=K  T_nominal_value=1  Q_specify=off  Q_priority=None  Q=0 W  Q_nominal_specify=off  Q_nominal_unit=W  Q_nominal_value=1
  Radiative Heat Transfer{,1..9} (10 alike) : fl_lib/Thermal/Thermal Elements/Radiative Heat Transfer  area=A_empty_b m^2  rad_tr_coeff=Gr_kap_mli W/(m^2*K^4)  T_specify=off  T_priority=None  T=0 K  T_nominal_specify=off  T_nominal_unit=K  T_nominal_value=1  Q_specify=off  Q_priority=None  Q=0 W  Q_nominal_specify=off  Q_nominal_unit=W  Q_nominal_value=1
      settings: SourceProductBaseCode=SS  InternalSimscapePortConfiguration="{\"Bottom\":[],\"Left\":[{\"id\":\"A\",\"label\":\"A\",\"type\":\"foundation.thermal.thermal\"}],\"Right\":[{\"id\":\"B\",\"label\":\"B\",\"type\":\"foundation.thermal.thermal\"}],\"Top\":[]}"
  Conn_DS : PMIOPort  Side=Right
  PL : PMIOPort  Port=2  Side=Left
  connections:
  Conductive Heat Transfer13/RConn1 -- Conductive Heat Transfer1/LConn1
  PL/RConn1 -- Conductive Heat Transfer13/LConn1
  Conductive Heat Transfer10/LConn1 -- Conductive Heat Transfer22/RConn1 -- Radiative Heat Transfer8/RConn1
  Conductive Heat Transfer9/RConn1 -- Conductive Heat Transfer22/LConn1 -- Radiative Heat Transfer8/LConn1
  Conductive Heat Transfer2/RConn1 -- Radiative Heat Transfer1/LConn1 -- Conductive Heat Transfer15/LConn1
  Conn_DS/RConn1 -- Conductive Heat Transfer23/RConn1 -- Radiative Heat Transfer9/RConn1
  Radiative Heat Transfer1/RConn1 -- Conductive Heat Transfer15/RConn1 -- Conductive Heat Transfer3/LConn1
  Conductive Heat Transfer4/LConn1 -- Conductive Heat Transfer16/RConn1 -- Radiative Heat Transfer2/RConn1
  Conductive Heat Transfer3/RConn1 -- Conductive Heat Transfer16/LConn1 -- Radiative Heat Transfer2/LConn1
  Conductive Heat Transfer2/LConn1 -- Conductive Heat Transfer14/RConn1 -- Radiative Heat Transfer/RConn1
  Conductive Heat Transfer10/RConn1 -- Conductive Heat Transfer23/LConn1 -- Radiative Heat Transfer9/LConn1
  Radiative Heat Transfer3/RConn1 -- Conductive Heat Transfer17/RConn1 -- Conductive Heat Transfer5/LConn1
  Conductive Heat Transfer6/LConn1 -- Radiative Heat Transfer4/RConn1 -- Conductive Heat Transfer18/RConn1
  Radiative Heat Transfer7/RConn1 -- Conductive Heat Transfer21/RConn1 -- Conductive Heat Transfer9/LConn1
  Radiative Heat Transfer6/LConn1 -- Conductive Heat Transfer20/LConn1 -- Conductive Heat Transfer7/RConn1
  Conductive Heat Transfer5/RConn1 -- Conductive Heat Transfer18/LConn1 -- Radiative Heat Transfer4/LConn1
  Conductive Heat Transfer14/LConn1 -- Conductive Heat Transfer1/RConn1 -- Radiative Heat Transfer/LConn1
  Conductive Heat Transfer7/LConn1 -- Conductive Heat Transfer19/RConn1 -- Radiative Heat Transfer5/RConn1
  Conductive Heat Transfer4/RConn1 -- Radiative Heat Transfer3/LConn1 -- Conductive Heat Transfer17/LConn1
  Conductive Heat Transfer8/RConn1 -- Radiative Heat Transfer7/LConn1 -- Conductive Heat Transfer21/LConn1
  Conductive Heat Transfer8/LConn1 -- Radiative Heat Transfer6/RConn1 -- Conductive Heat Transfer20/RConn1
  Conductive Heat Transfer6/RConn1 -- Radiative Heat Transfer5/LConn1 -- Conductive Heat Transfer19/LConn1

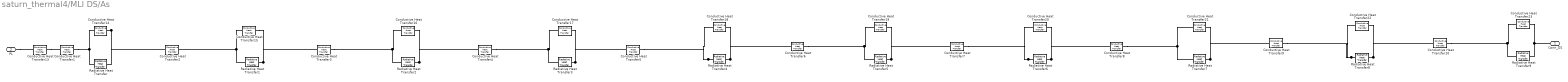
== system saturn_thermal4/MLI DS/As ==
  Conductive Heat Transfer{1..10} (10 alike) : fl_lib/Thermal/Thermal Elements/Conductive Heat Transfer  area=As m^2  thickness=s_kap m  th_cond=k_kap W/(m*K)  T_specify=off  T_priority=None  T=0 K  T_nominal_specify=off  T_nominal_unit=K  T_nominal_value=1  Q_specify=off  Q_priority=None  Q=0 W  Q_nominal_specify=off  Q_nominal_unit=W  Q_nominal_value=1
  Conductive Heat Transfer13 : fl_lib/Thermal/Thermal Elements/Conductive Heat Transfer  area=As m^2  thickness=s_al m  th_cond=k_al W/(m*K)  T_specify=off  T_priority=None  T=0 K  T_nominal_specify=off  T_nominal_unit=K  T_nominal_value=1  Q_specify=off  Q_priority=None  Q=0 W  Q_nominal_specify=off  Q_nominal_unit=W  Q_nominal_value=1
  Conductive Heat Transfer{14..23} (10 alike) : fl_lib/Thermal/Thermal Elements/Conductive Heat Transfer  area=A_net_new m^2  thickness=s_tfe_out m  th_cond=k_tfe W/(m*K)  T_specify=off  T_priority=None  T=0 K  T_nominal_specify=off  T_nominal_unit=K  T_nominal_value=1  Q_specify=off  Q_priority=None  Q=0 W  Q_nominal_specify=off  Q_nominal_unit=W  Q_nominal_value=1
  Radiative Heat Transfer{,1..9} (10 alike) : fl_lib/Thermal/Thermal Elements/Radiative Heat Transfer  area=A_empty m^2  rad_tr_coeff=Gr_kap_mli W/(m^2*K^4)  T_specify=off  T_priority=None  T=0 K  T_nominal_specify=off  T_nominal_unit=K  T_nominal_value=1  Q_specify=off  Q_priority=None  Q=0 W  Q_nominal_specify=off  Q_nominal_unit=W  Q_nominal_value=1
      settings: SourceProductBaseCode=SS  InternalSimscapePortConfiguration="{\"Bottom\":[],\"Left\":[{\"id\":\"A\",\"label\":\"A\",\"type\":\"foundation.thermal.thermal\"}],\"Right\":[{\"id\":\"B\",\"label\":\"B\",\"type\":\"foundation.thermal.thermal\"}],\"Top\":[]}"
  Conn_DS : PMIOPort  Side=Right
  PL : PMIOPort  Port=2  Side=Left
  connections:
  Radiative Heat Transfer5/LConn1 -- Conductive Heat Transfer19/LConn1 -- Conductive Heat Transfer6/RConn1
  Radiative Heat Transfer6/RConn1 -- Conductive Heat Transfer20/RConn1 -- Conductive Heat Transfer8/LConn1
  Conductive Heat Transfer21/LConn1 -- Conductive Heat Transfer8/RConn1 -- Radiative Heat Transfer7/LConn1
  Conductive Heat Transfer17/LConn1 -- Radiative Heat Transfer3/LConn1 -- Conductive Heat Transfer4/RConn1
  Radiative Heat Transfer5/RConn1 -- Conductive Heat Transfer19/RConn1 -- Conductive Heat Transfer7/LConn1
  Conductive Heat Transfer13/RConn1 -- Conductive Heat Transfer1/LConn1
  Radiative Heat Transfer4/LConn1 -- Conductive Heat Transfer18/LConn1 -- Conductive Heat Transfer5/RConn1
  Radiative Heat Transfer6/LConn1 -- Conductive Heat Transfer20/LConn1 -- Conductive Heat Transfer7/RConn1
  Radiative Heat Transfer7/RConn1 -- Conductive Heat Transfer21/RConn1 -- Conductive Heat Transfer9/LConn1
  Radiative Heat Transfer4/RConn1 -- Conductive Heat Transfer18/RConn1 -- Conductive Heat Transfer6/LConn1
  Radiative Heat Transfer3/RConn1 -- Conductive Heat Transfer17/RConn1 -- Conductive Heat Transfer5/LConn1
  Radiative Heat Transfer9/LConn1 -- Conductive Heat Transfer23/LConn1 -- Conductive Heat Transfer10/RConn1
  Conductive Heat Transfer14/RConn1 -- Radiative Heat Transfer/RConn1 -- Conductive Heat Transfer2/LConn1
  Radiative Heat Transfer2/LConn1 -- Conductive Heat Transfer16/LConn1 -- Conductive Heat Transfer3/RConn1
  Radiative Heat Transfer2/RConn1 -- Conductive Heat Transfer16/RConn1 -- Conductive Heat Transfer4/LConn1
  Radiative Heat Transfer1/RConn1 -- Conductive Heat Transfer15/RConn1 -- Conductive Heat Transfer3/LConn1
  Conductive Heat Transfer23/RConn1 -- Conn_DS/RConn1 -- Radiative Heat Transfer9/RConn1
  Conductive Heat Transfer15/LConn1 -- Radiative Heat Transfer1/LConn1 -- Conductive Heat Transfer2/RConn1
  Radiative Heat Transfer8/LConn1 -- Conductive Heat Transfer22/LConn1 -- Conductive Heat Transfer9/RConn1
  Radiative Heat Transfer8/RConn1 -- Conductive Heat Transfer22/RConn1 -- Conductive Heat Transfer10/LConn1
  PL/RConn1 -- Conductive Heat Transfer13/LConn1
  Conductive Heat Transfer1/RConn1 -- Conductive Heat Transfer14/LConn1 -- Radiative Heat Transfer/LConn1
